simulink model "copy"  (R2019b)
settings: Solver=VariableStepAuto  StartTime=0.0  StopTime=0.5  RelTol=1e-3
values from neighbouring files (symbols this model uses):
  bitRate = 250000    [ModemDesign6LoWPAN.m]
  cps = 32    [ModemDesign6LoWPAN.m]
undefined symbols (not defined in the file or in its folder): doppler, magnitude
libraries: dspmathops x3, commchan3 x2, commdigbbndpm3 x2, commutil2 x2, commrfcorlib x1, commsink2 x1, commrandsrc3 x1
settings Model: Creator=kaushik  LastModifiedBy=kaushik
settings DataIOCC: ReturnWorkspaceOutputs=off

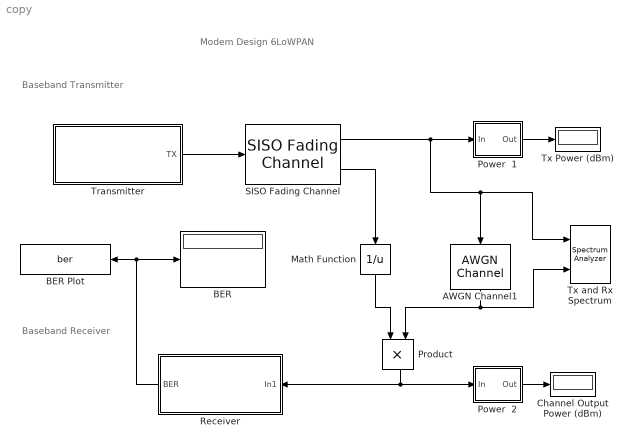
== system copy ==
  note: Modem Design 6LoWPAN
  note: Baseband Receiver
  note: Baseband Transmitter
  AWGN Channel1 : commchan3/AWGN Channel  InputProcessing=Columns as channels (frame based)  seed=73  noiseMode="Signal to noise ratio  (Eb/No)"  EbNodB=EbNo  EsNodB=-2.1  SNRdB=-2.7  bitsPerSym=1  Ps=1e-3*10^(-100/10)  Tsym="2/(bitRate)  % 2 bits per OQPSK symbol"  variance=1
      settings: SourceProductName=Communications Toolbox
  BER : Display
  BER Plot : ToWorkspace  VariableName=ber  SampleTime=-1
      settings: MaxDataPoints=2  Save2DSignal=2-D array (concatenate along first dimension)
  Channel Output Power (dBm) : Display
  Math Function : Math  Operator=reciprocal  SignedPower=off  SaturateOnIntegerOverflow=on
  Power  1 : Subsystem  mask{R=1}
      mask prompts: R "Reference Impedance [Ohm]"
      mask DialogControl DescGroupVar Prompt: Power Meter
      mask Display: disp('Power \nMeter')
  Power  2 : Subsystem  mask{R=1}
      mask prompts: R "Reference Impedance [Ohm]"
      mask DialogControl DescGroupVar Prompt: Power Meter
      mask Display: disp('Power \nMeter')
  Product : Product
  Receiver : Subsystem
      mask Display:
      | disp('IEEE 802.15\nReceiver')
      | port_label('output', 1, 'BER')
  SISO Fading Channel : commchan3/SISO Fading Channel  InheritSampleRate=on  SampleRate=1  PathDelays=0  AveragePathGains=0  NormalizePathGains=on  FadingDistribution=Rician  KFactor=2  DirectPathDopplerShift=0  DirectPathInitialPhase=0  MaximumDopplerShift=0.001  DopplerSpectrum=doppler('Jakes')  RandomStream=mt19937ar with seed  Seed=73  PathGainsOutputPort=on  ChannelFilterDelayOutputPort=off  SimulateUsing=Interpreted execution  Visualization=Off  PathsForDopplerDisplay=1  SamplesToDisplay=25%
      settings: SourceProductName=Communications Toolbox
  Transmitter : Subsystem
      mask Display: disp('IEEE 802.15\nTransmitter')
  Tx Power (dBm) : Display
  Tx and Rx Spectrum : SpectrumAnalyzer  NumInputPorts=2
  wires:
  Power  2/1(Out) -> Channel Output Power (dBm)/1
  AWGN Channel1/1 -> Tx and Rx Spectrum/2, Product/2
  Power  1/1(Out) -> Tx Power (dBm)/1
  Receiver/1(BER) -> BER Plot/1, BER/1
  Transmitter/1(TX) -> SISO Fading Channel/1
  SISO Fading Channel/1 -> Power  1/1(In), Tx and Rx Spectrum/1, AWGN Channel1/1
  SISO Fading Channel/2 -> Math Function/1
  Math Function/1 -> Product/1
  Product/1 -> Receiver/1(In1), Power  2/1(In)

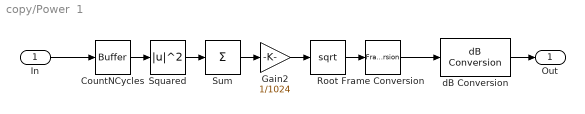
== system copy/Power  1 ==
  In : Inport
  CountNCycles : Buffer  N=1024
  Frame Conversion : FrameConversion  OutFrame=Sample-based
  Gain2 : Gain  Gain=1/1024
  Root : Sqrt  SaturateOnIntegerOverflow=on
  Squared : Math  Operator=magnitude^2  SaturateOnIntegerOverflow=on
  Sum : Sum  Inputs=+  CollapseMode=Specified dimension
  dB Conversion : dspmathops/dB Conversion  dBtype=dBm  intype=Amplitude  R=R  fuzz=on
      settings: SourceProductName=DSP System Toolbox
  Out : Outport  VectorParamsAs1DForOutWhenUnconnected=off
  wires:
  dB Conversion/1 -> Out/1
  In/1 -> CountNCycles/1
  Frame Conversion/1 -> dB Conversion/1
  CountNCycles/1 -> Squared/1
  Squared/1 -> Sum/1
  Sum/1 -> Gain2/1
  Root/1 -> Frame Conversion/1
  Gain2/1 -> Root/1

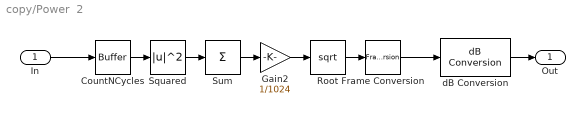
== system copy/Power  2 ==
  In : Inport
  CountNCycles : Buffer  N=1024
  Frame Conversion : FrameConversion  OutFrame=Sample-based
  Gain2 : Gain  Gain=1/1024
  Root : Sqrt  SaturateOnIntegerOverflow=on
  Squared : Math  Operator=magnitude^2  SaturateOnIntegerOverflow=on
  Sum : Sum  Inputs=+  CollapseMode=Specified dimension
  dB Conversion : dspmathops/dB Conversion  dBtype=dBm  intype=Amplitude  R=R  fuzz=on
      settings: SourceProductName=DSP System Toolbox
  Out : Outport  VectorParamsAs1DForOutWhenUnconnected=off
  wires:
  Gain2/1 -> Root/1
  Root/1 -> Frame Conversion/1
  Sum/1 -> Gain2/1
  Squared/1 -> Sum/1
  CountNCycles/1 -> Squared/1
  Frame Conversion/1 -> dB Conversion/1
  In/1 -> CountNCycles/1
  dB Conversion/1 -> Out/1

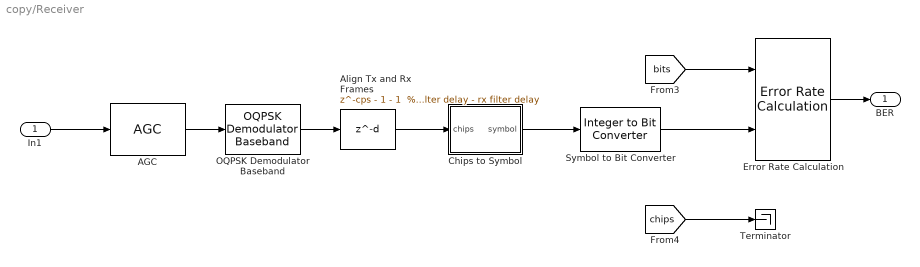
== system copy/Receiver ==
  In1 : Inport
  AGC : commrfcorlib/AGC  LegacyMode=off  DetectorMethod=Rectifier  LoopMethod=Linear  UpdatePeriod=100  StepSize=0.1  AdaptationStepSize=0.01  DesiredOutputPower=1  AveragingLength=100  MaximumGain=30  MaxPowerGain=200  GainOutputPort=off  InputPowerOutputPort=off  SimulateUsing=Interpreted execution
      settings: SourceProductName=Communications Toolbox
  Align Tx and Rx Frames : Delay  DelayLength="cps - 1 - 1  % chips/sym - tx filter delay - rx filter delay"  InputProcessing=Columns as channels (frame based)
  Chips to Symbol : MATLAB Function  TreatAsAtomicUnit=on
  Error Rate Calculation : commsink2/Error Rate Calculation  N=4  st_delay=0  cp_mode=Entire frame  subframe=[]  PMode=Port  WsName=ErrorVec  RsMode2=off  stop=on  numErr=100  maxBits=1e7
      settings: SourceProductName=Communications Toolbox
  OQPSK Demodulator Baseband : commdigbbndpm3/OQPSK Demodulator Baseband  OutType=Bit  Ph=0  Mapping=Gray  pulseShape=Half sine  num=[0.7071, 0.7071]  rolloff=1  filterSpan=10  sps=sps  RateOptions=Enforce single-rate processing  outDtype2=double
      settings: SourceProductName=Communications Toolbox  SourceProductBaseCode=CM
  Symbol to Bit Converter : commutil2/Integer to Bit Converter  nbits=4  signedInputValues=Unsigned  bitOrder=MSB first  outDtype=Inherit via internal rule
      settings: SourceProductName=Communications Toolbox
  Terminator : Terminator
  BER : Outport  VectorParamsAs1DForOutWhenUnconnected=off
  wires:
  In1/1 -> AGC/1
  Error Rate Calculation/1 -> BER/1
  [bits] -> Error Rate Calculation/1
  [chips] -> Terminator/1
  Align Tx and Rx Frames/1 -> Chips to Symbol/1(chips)
  Chips to Symbol/1(symbol) -> Symbol to Bit Converter/1
  OQPSK Demodulator Baseband/1 -> Align Tx and Rx Frames/1
  AGC/1 -> OQPSK Demodulator Baseband/1
  Symbol to Bit Converter/1 -> Error Rate Calculation/2

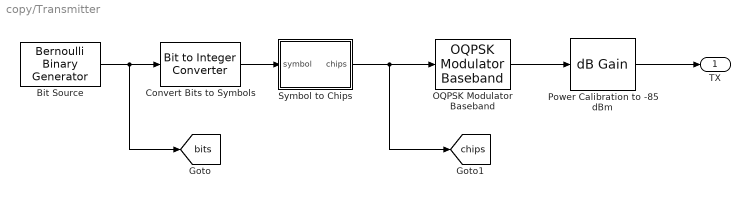
== system copy/Transmitter ==
  Bit Source : commrandsrc3/Bernoulli Binary Generator  ProbabilityOfZero=0.5  SeedSource=Parameter  Seed=73  SampleTime=1/bitRate  SamplesPerFrame=bitsPerFrame  OutputDataType=double  SimulateUsing=Interpreted execution
      settings: SourceProductName=Communications Toolbox
  Convert Bits to Symbols : commutil2/Bit to Integer Converter  nbits=4  bitOrder=MSB first  signedOutputValues=Unsigned  outDtype=Inherit via internal rule  outDtypeSigned=Inherit via internal rule
      settings: SourceProductName=Communications Toolbox
  OQPSK Modulator Baseband : commdigbbndpm3/OQPSK Modulator Baseband  InType=Bit  Ph=0  Mapping=Gray  pulseShape=Half sine  num=[0.7071, 0.7071]  rolloff=1  filterSpan=10  sps=sps  RateOptions=Enforce single-rate processing  outDtype=double
      settings: SourceProductName=Communications Toolbox  SourceProductBaseCode=CM
  Power Calibration to -85 dBm : dspmathops/dB Gain  dB=-118.159 % power of preceding block is 1 W  intype=Amplitude
      settings: SourceProductName=DSP System Toolbox  SourceProductBaseCode=DS
  Symbol to Chips : MATLAB Function  TreatAsAtomicUnit=on
  TX : Outport
  tag scope: bits=global, chips=global
  wires:
  Power Calibration to -85 dBm/1 -> TX/1
  Symbol to Chips/1(chips) -> OQPSK Modulator Baseband/1, [chips]
  Convert Bits to Symbols/1 -> Symbol to Chips/1(symbol)
  OQPSK Modulator Baseband/1 -> Power Calibration to -85 dBm/1
  Bit Source/1 -> [bits], Convert Bits to Symbols/1

== matlab function copy/Receiver/Chips to Symbol ==
  data: chips input; symbol output size=[1 1]
function symbol = chips2sym(chips)
  chipMap = ...
     [1 1 0 1 1 0 0 1 1 1 0 0 0 0 1 1 0 1 0 1 0 0 1 0 0 0 1 0 1 1 1 0;
      1 1 1 0 1 1 0 1 1 0 0 1 1 1 0 0 0 0 1 1 0 1 0 1 0 0 1 0 0 0 1 0;
      0 0 1 0 1 1 1 0 1 1 0 1 1 0 0 1 1 1 0 0 0 0 1 1 0 1 0 1 0 0 1 0;
      0 0 1 0 0 0 1 0 1 1 1 0 1 1 0 1 1 0 0 1 1 1 0 0 0 0 1 1 0 1 0 1;
      0 1 0 1 0 0 1 0 0 0 1 0 1 1 1 0 1 1 0 1 1 0 0 1 1 1 0 0 0 0 1 1;
      0 0 1 1 0 1 0 1 0 0 1 0 0 0 1 0 1 1 1 0 1 1 0 1 1 0 0 1 1 1 0 0;
      1 1 0 0 0 0 1 1 0 1 0 1 0 0 1 0 0 0 1 0 1 1 1 0 1 1 0 1 1 0 0 1;
      1 0 0 1 1 1 0 0 0 0 1 1 0 1 0 1 0 0 1 0 0 0 1 0 1 1 1 0 1 1 0 1;
      1 0 0 0 1 1 0 0 1 0 0 1 0 1 1 0 0 0 0 0 0 1 1 1 0 1 1 1 1 0 1 1;
      1 0 1 1 1 0 0 0 1 1 0 0 1 0 0 1 0 1 1 0 0 0 0 0 0 1 1 1 0 1 1 1;
      0 1 1 1 1 0 1 1 1 0 0 0 1 1 0 0 1 0 0 1 0 1 1 0 0 0 0 0 0 1 1 1;
      0 1 1 1 0 1 1 1 1 0 1 1 1 0 0 0 1 1 0 0 1 0 0 1 0 1 1 0 0 0 0 0;
      0 0 0 0 0 1 1 1 0 1 1 1 1 0 1 1 1 0 0 0 1 1 0 0 1 0 0 1 0 1 1 0;
      0 1 1 0 0 0 0 0 0 1 1 1 0 1 1 1 1 0 1 1 1 0 0 0 1 1 0 0 1 0 0 1;
      1 0 0 1 0 1 1 0 0 0 0 0 0 1 1 1 0 1 1 1 1 0 1 1 1 0 0 0 1 1 0 0;
      1 1 0 0 1 0 0 1 0 1 1 0 0 0 0 0 0 1 1 1 0 1 1 1 1 0 1 1 1 0 0 0];

numSeq = size(chipMap, 1);
repChips = repmat(chips, 1, numSeq);
despreadOut = sum(abs(repChips - chipMap'));
[~, symIdx] = min(despreadOut);
symbol = symIdx - 1;  % Convert from 1-based to 0-based indexing

== matlab function copy/Transmitter/Symbol to Chips ==
  data: symbol input; chips output size=[32 1]
function chips = sym2chips(symbol)
  chipMap = ...
     [1 1 0 1 1 0 0 1 1 1 0 0 0 0 1 1 0 1 0 1 0 0 1 0 0 0 1 0 1 1 1 0;
      1 1 1 0 1 1 0 1 1 0 0 1 1 1 0 0 0 0 1 1 0 1 0 1 0 0 1 0 0 0 1 0;
      0 0 1 0 1 1 1 0 1 1 0 1 1 0 0 1 1 1 0 0 0 0 1 1 0 1 0 1 0 0 1 0;
      0 0 1 0 0 0 1 0 1 1 1 0 1 1 0 1 1 0 0 1 1 1 0 0 0 0 1 1 0 1 0 1;
      0 1 0 1 0 0 1 0 0 0 1 0 1 1 1 0 1 1 0 1 1 0 0 1 1 1 0 0 0 0 1 1;
      0 0 1 1 0 1 0 1 0 0 1 0 0 0 1 0 1 1 1 0 1 1 0 1 1 0 0 1 1 1 0 0;
      1 1 0 0 0 0 1 1 0 1 0 1 0 0 1 0 0 0 1 0 1 1 1 0 1 1 0 1 1 0 0 1;
      1 0 0 1 1 1 0 0 0 0 1 1 0 1 0 1 0 0 1 0 0 0 1 0 1 1 1 0 1 1 0 1;
      1 0 0 0 1 1 0 0 1 0 0 1 0 1 1 0 0 0 0 0 0 1 1 1 0 1 1 1 1 0 1 1;
      1 0 1 1 1 0 0 0 1 1 0 0 1 0 0 1 0 1 1 0 0 0 0 0 0 1 1 1 0 1 1 1;
      0 1 1 1 1 0 1 1 1 0 0 0 1 1 0 0 1 0 0 1 0 1 1 0 0 0 0 0 0 1 1 1;
      0 1 1 1 0 1 1 1 1 0 1 1 1 0 0 0 1 1 0 0 1 0 0 1 0 1 1 0 0 0 0 0;
      0 0 0 0 0 1 1 1 0 1 1 1 1 0 1 1 1 0 0 0 1 1 0 0 1 0 0 1 0 1 1 0;
      0 1 1 0 0 0 0 0 0 1 1 1 0 1 1 1 1 0 1 1 1 0 0 0 1 1 0 0 1 0 0 1;
      1 0 0 1 0 1 1 0 0 0 0 0 0 1 1 1 0 1 1 1 1 0 1 1 1 0 0 0 1 1 0 0;
      1 1 0 0 1 0 0 1 0 1 1 0 0 0 0 0 0 1 1 1 0 1 1 1 1 0 1 1 1 0 0 0];

 chips = chipMap(1+symbol,:)'; % +1 for 1-based indexing
